simulink model "AcasXuClosedLoop_m_1"  (R2019b)
settings: Solver=VariableStepAuto  StartTime=0.0  StopTime=30  RelTol=1e-3
libraries: neural x1560, simulink x2
(part 3 of 85)

== system AcasXuClosedLoop_m_1/networks/AcasXu_2_1/Process Output 1 ==
  a : Inport  PortDimensions=5
      mask Display: e = 0.06;c1 = [120 230 180]/255;c2 = ([120 230 180]+0)/(256+128);c3 = ([120 230 180]+128)/(256+128);patch([0 1 1 0],[0 0 1 1],c1);patch([0 1 1 1-e 1-e 0+e],[0 0 1 1-e 0+e 0+e],c2);patch([0 0 1 1-e 0+e 0+e],[0 1 1 1-e 1-e 0+e],c3);plot([0 1 1 0 0],[0 0 1 1 0]);
  y : Outport  PortDimensions=5
      mask Display: e = 0.06;c1 = [120 230 180]/255;c2 = ([120 230 180]+0)/(256+128);c3 = ([120 230 180]+128)/(256+128);patch([0 1 1 0],[0 0 1 1],c1);patch([0 1 1 1-e 1-e 0+e],[0 0 1 1-e 0+e 0+e],c2);patch([0 0 1 1-e 0+e 0+e],[0 1 1 1-e 1-e 0+e],c3);plot([0 1 1 0 0],[0 0 1 1 0]);
  wires:
  a/1 -> y/1

== system AcasXuClosedLoop_m_1/networks/AcasXu_3_1/Layer 1 ==
  "p{1}" : Inport  PortDimensions=5
      mask Display: e = 0.06;c1 = [120 230 180]/255;c2 = ([120 230 180]+0)/(256+128);c3 = ([120 230 180]+128)/(256+128);patch([0 1 1 0],[0 0 1 1],c1);patch([0 1 1 1-e 1-e 0+e],[0 0 1 1-e 0+e 0+e],c2);patch([0 0 1 1-e 0+e 0+e],[0 1 1 1-e 1-e 0+e],c3);plot([0 1 1 0 0],[0 0 1 1 0]);
  Delays 1 : Subsystem
      mask Display: e = 0.06;c1 = [120 150 230]/255;c2 = ([120 150 230]+0)/383;c3 = ([120 150 230]+128)/383;patch([0 1 1 0],[0 0 1 1],c1);patch([0 1 1 1-e 1-e 0+e],[0 0 1 1-e 0+e 0+e],c2);patch([0 0 1 1-e 0+e 0+e],[0 1 1 1-e 1-e 0+e],c3);plot([0 1 1 0 0],[0 0 1 1 0]);disp('0');
  "IW{1,1}" : Subsystem
      mask Display: e = 0.06;c1 = [120 150 230]/255;c2 = ([120 150 230]+0)/383;c3 = ([120 150 230]+128)/383;patch([0 1 1 0],[0 0 1 1],c1);patch([0 1 1 1-e 1-e 0+e],[0 0 1 1-e 0+e 0+e],c2);patch([0 0 1 1-e 0+e 0+e],[0 1 1 1-e 1-e 0+e],c3);plot([0 1 1 0 0],[0 0 1 1 0]);disp('W');
  "b{1}" : Constant  Value=[-0.63411600000000001298161578233703039586544036865234375;-0.86285800000000001386268877467955462634563446044921875;0.0263649000000000001409095062854248681105673313140869140625;-0.77790700000000001512745484433253295719623565673828125;-0.172433000000000002938094212368014268577098846435546875;0.08491990000000000649027498411669512279331684112548828125;0.2125950000000000061906035853098728694021701812744140625;-0.0674716999999999955672791429606149904429912567138671875;-0.37667200000000000681410483593936078250408172607421875;0.2037360000000000004316547119742608629167079925537109375;0.1262359999999999871089784164723823778331279754638671875;-0.5560300000000000242295072894194163382053375244140625;-0.45896700000000001384847791996435262262821197509765625;-0.306524000000000018673063095775432884693145751953125;-0.06648220000000000518003417937507038004696369171142578125;-0.53795800000000004725819735540426336228847503662109375;0.3475610000000000088249407781404443085193634033203125;-0.0226518999999999991190602344204307883046567440032958984375;-0.387670000000000014583889651476056315004825592041015625;-0.5660089999999999843538489585625939071178436279296875;-0.072275699999999998279776036724797450006008148193359375;0.1934430000000000038351544162651407532393932342529296875;0.16017300000000000981259518084698356688022613525390625;-0.11682399999999999729016764149491791613399982452392578125;0.0849908000000000052320814347694977186620235443115234375;-0.0176456000000000008676170892840673332102596759796142578125;-0.19644600000000000949995637711253948509693145751953125;0.193624999999999991562305012848810292780399322509765625;-0.6789519999999999999573674358543939888477325439453125;-0.045666199999999997072297475142477196641266345977783203125;0.1721910000000000107167608121017110534012317657470703125;-0.36496099999999997987032429591636173427104949951171875;-0.34974600000000000132871491587138734757900238037109375;-0.56786199999999997789501549050328321754932403564453125;-0.770345999999999975216269376687705516815185546875;-0.10563799999999999579269882588050677441060543060302734375;-0.82683600000000001539746108392137102782726287841796875;0.5441249999999999698019337301957421004772186279296875;0.552065999999999945657691569067537784576416015625;-0.279227999999999976221687347788247279822826385498046875;-0.0244107999999999998597122186083652195520699024200439453125;-0.6494180000000000507753838974167592823505401611328125;-0.67569800000000002082600758512853644788265228271484375;-0.0534702999999999983860021757209324277937412261962890625;0.043996899999999998509547793901219847612082958221435546875;-0.10106999999999999317878973670303821563720703125;0.10270100000000000062261307220978778786957263946533203125;0.385166999999999981607601284849806688725948333740234375;-0.642935000000000034248159863636828958988189697265625;-0.0231879000000000008718803456986279343254864215850830078125]
      mask Display: e = 0.06;c1 = [120 150 230]/255;c2 = ([120 150 230]+0)/383;c3 = ([120 150 230]+128)/383;patch([0 1 1 0],[0 0 1 1],c1);patch([0 1 1 1-e 1-e 0+e],[0 0 1 1-e 0+e 0+e],c2);patch([0 0 1 1-e 0+e 0+e],[0 1 1 1-e 1-e 0+e],c3);plot([0 1 1 0 0],[0 0 1 1 0]);disp('b');
  netsum : Sum  Inputs=2  SaturateOnIntegerOverflow=on  InputSameDT=on  OutDataTypeStr=Inherit: Same as first input
      mask Display: e = 0.06;c1 = [120 150 230]/255;c2 = ([120 150 230]+0)/383;c3 = ([120 150 230]+128)/383;patch([0 1 1 0],[0 0 1 1],c1);patch([0 1 1 1-e 1-e 0+e],[0 0 1 1-e 0+e 0+e],c2);patch([0 0 1 1-e 0+e 0+e],[0 1 1 1-e 1-e 0+e],c3);plot([0 1 1 0 0],[0 0 1 1 0]);disp('+');
  tansig : neural/Transfer Functions/tansig
      settings: SourceProductName=Deep Learning Toolbox
  "a{1}" : Outport  InitialOutput=[0;0;0;0;0;0;0;0;0;0;0;0;0;0;0;0;0;0;0;0;0;0;0;0;0;0;0;0;0;0;0;0;0;0;0;0;0;0;0;0;0;0;0;0;0;0;0;0;0;0]
      mask Display: e = 0.06;c1 = [120 230 180]/255;c2 = ([120 230 180]+0)/(256+128);c3 = ([120 230 180]+128)/(256+128);patch([0 1 1 0],[0 0 1 1],c1);patch([0 1 1 1-e 1-e 0+e],[0 0 1 1-e 0+e 0+e],c2);patch([0 0 1 1-e 0+e 0+e],[0 1 1 1-e 1-e 0+e],c3);plot([0 1 1 0 0],[0 0 1 1 0]);
  wires:
  tansig/1 -> "a{1}"/1
  netsum/1 -> tansig/1
  "b{1}"/1 -> netsum/2
  "IW{1,1}"/1("iz{1,1}") -> netsum/1
  Delays 1/1("pd{1,1}") -> "IW{1,1}"/1("pd{1,1}")
  "p{1}"/1 -> Delays 1/1("p{1}")

== system AcasXuClosedLoop_m_1/networks/AcasXu_3_1/Layer 2 ==
  "a{1} " : Inport  PortDimensions=50
      mask Display: e = 0.06;c1 = [120 230 180]/255;c2 = ([120 230 180]+0)/(256+128);c3 = ([120 230 180]+128)/(256+128);patch([0 1 1 0],[0 0 1 1],c1);patch([0 1 1 1-e 1-e 0+e],[0 0 1 1-e 0+e 0+e],c2);patch([0 0 1 1-e 0+e 0+e],[0 1 1 1-e 1-e 0+e],c3);plot([0 1 1 0 0],[0 0 1 1 0]);
  Delays 1 : Subsystem
      mask Display: e = 0.06;c1 = [120 150 230]/255;c2 = ([120 150 230]+0)/383;c3 = ([120 150 230]+128)/383;patch([0 1 1 0],[0 0 1 1],c1);patch([0 1 1 1-e 1-e 0+e],[0 0 1 1-e 0+e 0+e],c2);patch([0 0 1 1-e 0+e 0+e],[0 1 1 1-e 1-e 0+e],c3);plot([0 1 1 0 0],[0 0 1 1 0]);disp('0');
  "LW{2,1}" : Subsystem
      mask Display: e = 0.06;c1 = [120 150 230]/255;c2 = ([120 150 230]+0)/383;c3 = ([120 150 230]+128)/383;patch([0 1 1 0],[0 0 1 1],c1);patch([0 1 1 1-e 1-e 0+e],[0 0 1 1-e 0+e 0+e],c2);patch([0 0 1 1-e 0+e 0+e],[0 1 1 1-e 1-e 0+e],c3);plot([0 1 1 0 0],[0 0 1 1 0]);disp('W');
  "b{2}" : Constant  Value=[-0.421233000000000024076740601230994798243045806884765625;0.1434140000000000136903821612577303312718868255615234375;-0.99709400000000003583267016438185237348079681396484375;0.377188000000000023259616455106879584491252899169921875;-0.01035819999999999969919617370806008693762123584747314453125;-0.71935300000000002018651912294444628059864044189453125;-0.334293000000000006810552122260560281574726104736328125;-0.773163999999999962398078423575498163700103759765625;-0.003741040000000000163848934420229852548800408840179443359375;-0.0589896000000000031437963343705632723867893218994140625;-0.35057199999999999473487832801765762269496917724609375;-0.91174900000000003164046802339726127684116363525390625;-0.57765400000000000080291329140891321003437042236328125;-1.0581300000000000149924517245381139218807220458984375;0.278627000000000013546497257266310043632984161376953125;-0.0093275500000000004241496043277948047034442424774169921875;-0.0123510000000000008668621376273222267627716064453125;-0.404268000000000016225243371081887744367122650146484375;-0.746971999999999969332975524594075977802276611328125;-0.08297960000000000058140159353570197708904743194580078125;-1.167079999999999895266000748961232602596282958984375;-0.5178279999999999549942231169552542269229888916015625;0.68078300000000002700772938624140806496143341064453125;-0.2080639999999999989466203942356514744460582733154296875;-0.80007799999999995588240153665537945926189422607421875;5.53026000000000013986749258787511962509597651660442352294921875e-05;-0.1960199999999999997957189634689711965620517730712890625;0.600638000000000005229594535194337368011474609375;0.28952699999999997881872104699141345918178558349609375;0.48111599999999998811262003073352389037609100341796875;0.028625799999999999856381549534489749930799007415771484375;0.255568999999999990624388601645478047430515289306640625;-0.00619316999999999957815521867132702027447521686553955078125;-0.7419949999999999601385525238583795726299285888671875;-0.1441759999999999986020071673920028842985630035400390625;-0.556777999999999995139887687400914728641510009765625;-0.2580999999999999960920149533194489777088165283203125;-0.282907999999999992812860227786586619913578033447265625;-0.48276499999999999968025576890795491635799407958984375;-0.004546970000000000004802824804528427193872630596160888671875;0.302254999999999995896615700985421426594257354736328125;-0.6570489999999999941593387120519764721393585205078125;-0.5748919999999999586037802146165631711483001708984375;1.2579299999999999926103555480949580669403076171875;0.222015999999999991132426657713949680328369140625;1.349930000000000074322770160506479442119598388671875;-0.423561000000000020815349444092134945094585418701171875;-0.427883000000000013329781722859479486942291259765625;0.304840999999999973102404737801407463848590850830078125;-0.10981899999999999995026200849679298698902130126953125]
      mask Display: e = 0.06;c1 = [120 150 230]/255;c2 = ([120 150 230]+0)/383;c3 = ([120 150 230]+128)/383;patch([0 1 1 0],[0 0 1 1],c1);patch([0 1 1 1-e 1-e 0+e],[0 0 1 1-e 0+e 0+e],c2);patch([0 0 1 1-e 0+e 0+e],[0 1 1 1-e 1-e 0+e],c3);plot([0 1 1 0 0],[0 0 1 1 0]);disp('b');
  netsum : Sum  Inputs=2  SaturateOnIntegerOverflow=on  InputSameDT=on  OutDataTypeStr=Inherit: Same as first input
      mask Display: e = 0.06;c1 = [120 150 230]/255;c2 = ([120 150 230]+0)/383;c3 = ([120 150 230]+128)/383;patch([0 1 1 0],[0 0 1 1],c1);patch([0 1 1 1-e 1-e 0+e],[0 0 1 1-e 0+e 0+e],c2);patch([0 0 1 1-e 0+e 0+e],[0 1 1 1-e 1-e 0+e],c3);plot([0 1 1 0 0],[0 0 1 1 0]);disp('+');
  tansig : neural/Transfer Functions/tansig
      settings: SourceProductName=Deep Learning Toolbox
  "a{2}" : Outport  InitialOutput=[0;0;0;0;0;0;0;0;0;0;0;0;0;0;0;0;0;0;0;0;0;0;0;0;0;0;0;0;0;0;0;0;0;0;0;0;0;0;0;0;0;0;0;0;0;0;0;0;0;0]
      mask Display: e = 0.06;c1 = [120 230 180]/255;c2 = ([120 230 180]+0)/(256+128);c3 = ([120 230 180]+128)/(256+128);patch([0 1 1 0],[0 0 1 1],c1);patch([0 1 1 1-e 1-e 0+e],[0 0 1 1-e 0+e 0+e],c2);patch([0 0 1 1-e 0+e 0+e],[0 1 1 1-e 1-e 0+e],c3);plot([0 1 1 0 0],[0 0 1 1 0]);
  wires:
  tansig/1 -> "a{2}"/1
  netsum/1 -> tansig/1
  "b{2}"/1 -> netsum/2
  "LW{2,1}"/1("lz{2,1}") -> netsum/1
  Delays 1/1("pd{2,1}") -> "LW{2,1}"/1("ad{2,1}")
  "a{1} "/1 -> Delays 1/1("p{2}")

== system AcasXuClosedLoop_m_1/networks/AcasXu_3_1/Layer 3 ==
  "a{2} " : Inport  PortDimensions=50
      mask Display: e = 0.06;c1 = [120 230 180]/255;c2 = ([120 230 180]+0)/(256+128);c3 = ([120 230 180]+128)/(256+128);patch([0 1 1 0],[0 0 1 1],c1);patch([0 1 1 1-e 1-e 0+e],[0 0 1 1-e 0+e 0+e],c2);patch([0 0 1 1-e 0+e 0+e],[0 1 1 1-e 1-e 0+e],c3);plot([0 1 1 0 0],[0 0 1 1 0]);
  Delays 1 : Subsystem
      mask Display: e = 0.06;c1 = [120 150 230]/255;c2 = ([120 150 230]+0)/383;c3 = ([120 150 230]+128)/383;patch([0 1 1 0],[0 0 1 1],c1);patch([0 1 1 1-e 1-e 0+e],[0 0 1 1-e 0+e 0+e],c2);patch([0 0 1 1-e 0+e 0+e],[0 1 1 1-e 1-e 0+e],c3);plot([0 1 1 0 0],[0 0 1 1 0]);disp('0');
  "LW{3,2}" : Subsystem
      mask Display: e = 0.06;c1 = [120 150 230]/255;c2 = ([120 150 230]+0)/383;c3 = ([120 150 230]+128)/383;patch([0 1 1 0],[0 0 1 1],c1);patch([0 1 1 1-e 1-e 0+e],[0 0 1 1-e 0+e 0+e],c2);patch([0 0 1 1-e 0+e 0+e],[0 1 1 1-e 1-e 0+e],c3);plot([0 1 1 0 0],[0 0 1 1 0]);disp('W');
  "b{3}" : Constant  Value=[1.0556000000000000937916411203332245349884033203125;-1.4562500000000000444089209850062616169452667236328125;0.35456500000000001904254531837068498134613037109375;-0.37268800000000001926281356645631603896617889404296875;1.9437599999999999322852772820624522864818572998046875;0.485267999999999977145392904276377521455287933349609375;-0.03026600000000000123545618180287419818341732025146484375;0.1490809999999999913011805574569734744727611541748046875;-1.6594700000000000006394884621840901672840118408203125;1.188099999999999933919525574310682713985443115234375;-1.2918600000000000083133500083931721746921539306640625;-0.263782000000000016459722473882720805704593658447265625;-0.73707800000000001094946355806314386427402496337890625;-0.85128499999999995839772282124613411724567413330078125;0.11599900000000000488409312993098865263164043426513671875;-0.062371299999999997576427546164268278516829013824462890625;-0.032435600000000001930100523850342142395675182342529296875;0.269172000000000022357227180691552348434925079345703125;-0.1436570000000000069118044621063745580613613128662109375;0.1983350000000000112887477143885917030274868011474609375;-1.749470000000000080575546235195361077785491943359375;-0.259944000000000008387956995647982694208621978759765625;-0.6662820000000000408846290156361646950244903564453125;0.1677220000000000099671382258748053573071956634521484375;-0.40030500000000002192024339819909073412418365478515625;-0.58646100000000001006839056572061963379383087158203125;-0.0123961999999999995802912877707058214582502841949462890625;-0.27758599999999999941024952931911684572696685791015625;0.322699000000000013610446103484719060361385345458984375;0.289306000000000007599254558954271487891674041748046875;-0.0636571999999999971198150205964338965713977813720703125;0.07619430000000000646753761657237191684544086456298828125;-0.26723200000000002507505314497393555939197540283203125;-0.886967999999999978655296217766590416431427001953125;0.074126899999999995571897670743055641651153564453125;-0.60304100000000004921929530610213987529277801513671875;-1.47614000000000000767386154620908200740814208984375;-0.99038400000000004208544623907073400914669036865234375;0.2862970000000000236894948102417401969432830810546875;0.01722970000000000057038818113142042420804500579833984375;-0.0288367999999999992388755032379776821471750736236572265625;0.55647699999999999942446038403431884944438934326171875;0.350275999999999976264319911933853290975093841552734375;-2.10245000000000015205614545266143977642059326171875;-0.0292092000000000011350476114557750406675040721893310546875;0.05668299999999999727595678677971591241657733917236328125;-0.7748880000000000212168060897965915501117706298828125;-0.030838999999999998358202191184318508021533489227294921875;-0.3683710000000000039932501749717630445957183837890625;-0.0617846999999999979547027351145516149699687957763671875]
      mask Display: e = 0.06;c1 = [120 150 230]/255;c2 = ([120 150 230]+0)/383;c3 = ([120 150 230]+128)/383;patch([0 1 1 0],[0 0 1 1],c1);patch([0 1 1 1-e 1-e 0+e],[0 0 1 1-e 0+e 0+e],c2);patch([0 0 1 1-e 0+e 0+e],[0 1 1 1-e 1-e 0+e],c3);plot([0 1 1 0 0],[0 0 1 1 0]);disp('b');
  netsum : Sum  Inputs=2  SaturateOnIntegerOverflow=on  InputSameDT=on  OutDataTypeStr=Inherit: Same as first input
      mask Display: e = 0.06;c1 = [120 150 230]/255;c2 = ([120 150 230]+0)/383;c3 = ([120 150 230]+128)/383;patch([0 1 1 0],[0 0 1 1],c1);patch([0 1 1 1-e 1-e 0+e],[0 0 1 1-e 0+e 0+e],c2);patch([0 0 1 1-e 0+e 0+e],[0 1 1 1-e 1-e 0+e],c3);plot([0 1 1 0 0],[0 0 1 1 0]);disp('+');
  tansig : neural/Transfer Functions/tansig
      settings: SourceProductName=Deep Learning Toolbox
  "a{3}" : Outport  InitialOutput=[0;0;0;0;0;0;0;0;0;0;0;0;0;0;0;0;0;0;0;0;0;0;0;0;0;0;0;0;0;0;0;0;0;0;0;0;0;0;0;0;0;0;0;0;0;0;0;0;0;0]
      mask Display: e = 0.06;c1 = [120 230 180]/255;c2 = ([120 230 180]+0)/(256+128);c3 = ([120 230 180]+128)/(256+128);patch([0 1 1 0],[0 0 1 1],c1);patch([0 1 1 1-e 1-e 0+e],[0 0 1 1-e 0+e 0+e],c2);patch([0 0 1 1-e 0+e 0+e],[0 1 1 1-e 1-e 0+e],c3);plot([0 1 1 0 0],[0 0 1 1 0]);
  wires:
  tansig/1 -> "a{3}"/1
  netsum/1 -> tansig/1
  "b{3}"/1 -> netsum/2
  "LW{3,2}"/1("lz{3,2}") -> netsum/1
  Delays 1/1("pd{3,2}") -> "LW{3,2}"/1("ad{3,2}")
  "a{2} "/1 -> Delays 1/1("p{3}")

== system AcasXuClosedLoop_m_1/networks/AcasXu_3_1/Layer 4 ==
  "a{3} " : Inport  PortDimensions=50
      mask Display: e = 0.06;c1 = [120 230 180]/255;c2 = ([120 230 180]+0)/(256+128);c3 = ([120 230 180]+128)/(256+128);patch([0 1 1 0],[0 0 1 1],c1);patch([0 1 1 1-e 1-e 0+e],[0 0 1 1-e 0+e 0+e],c2);patch([0 0 1 1-e 0+e 0+e],[0 1 1 1-e 1-e 0+e],c3);plot([0 1 1 0 0],[0 0 1 1 0]);
  Delays 1 : Subsystem
      mask Display: e = 0.06;c1 = [120 150 230]/255;c2 = ([120 150 230]+0)/383;c3 = ([120 150 230]+128)/383;patch([0 1 1 0],[0 0 1 1],c1);patch([0 1 1 1-e 1-e 0+e],[0 0 1 1-e 0+e 0+e],c2);patch([0 0 1 1-e 0+e 0+e],[0 1 1 1-e 1-e 0+e],c3);plot([0 1 1 0 0],[0 0 1 1 0]);disp('0');
  "LW{4,3}" : Subsystem
      mask Display: e = 0.06;c1 = [120 150 230]/255;c2 = ([120 150 230]+0)/383;c3 = ([120 150 230]+128)/383;patch([0 1 1 0],[0 0 1 1],c1);patch([0 1 1 1-e 1-e 0+e],[0 0 1 1-e 0+e 0+e],c2);patch([0 0 1 1-e 0+e 0+e],[0 1 1 1-e 1-e 0+e],c3);plot([0 1 1 0 0],[0 0 1 1 0]);disp('W');
  "b{4}" : Constant  Value=[0.1965349999999999874855660664252354763448238372802734375;-0.39496500000000001051603248924948275089263916015625;0.0831124000000000029420021974146948195993900299072265625;-0.8129589999999999871960199016029946506023406982421875;-0.267452999999999996294519633011077530682086944580078125;-0.62282899999999996598631923916400410234928131103515625;-0.5259570000000000078443918027915060520172119140625;0.16539300000000001222844048243132419884204864501953125;-1.460080000000000044479975258582271635532379150390625;2.108870000000000022311041902867145836353302001953125;-0.7184180000000000010373923942097462713718414306640625;0.334618999999999999772626324556767940521240234375;-0.0290208999999999987806642565146830747835338115692138671875;-1.4232800000000001006128513836301863193511962890625;0.1955969999999999930917482515724259428679943084716796875;0.2019459999999999866293620698343147523701190948486328125;-1.14275999999999999801048033987171947956085205078125;2.440440000000000164703806149191223084926605224609375;-0.0841351999999999933255168116374989040195941925048828125;-1.0137799999999999034372422102023847401142120361328125;0.919775000000000009237055564881302416324615478515625;-1.3366100000000000758149099056026898324489593505859375;-2.752540000000000208757455766317434608936309814453125;-0.10592500000000000526245713672324200160801410675048828125;-0.97771799999999997599076095866621471941471099853515625;0.3647489999999999898960822974913753569126129150390625;0.9579910000000000369624331142404116690158843994140625;-0.467220000000000024176216584237408824265003204345703125;0.09166290000000000548485701301615335978567600250244140625;-1.423890000000000100044417195022106170654296875;-1.8000700000000000589039927945123054087162017822265625;0.9487229999999999829896069059032015502452850341796875;-0.197079000000000004177991286269389092922210693359375;0.6932519999999999793516280988114885985851287841796875;-1.2097599999999999464961319972644560039043426513671875;-1.24059000000000008157030606525950133800506591796875;-0.63907999999999998141930745987338013947010040283203125;0.0181432000000000016870504992994028725661337375640869140625;-0.2202240000000000030855318300382350571453571319580078125;-1.83692000000000010828671292983926832675933837890625;2.902439999999999908908421275555156171321868896484375;0.259921999999999986386001182836480438709259033203125;0.74938099999999996381205846773809753358364105224609375;0.0329962000000000033050895353881060145795345306396484375;0.0563639999999999974367170807454385794699192047119140625;-1.997370000000000089812601800076663494110107421875;-0.378624999999999989341858963598497211933135986328125;0.5712930000000000507753838974167592823505401611328125;1.9845200000000000617461637375527061522006988525390625;0.39603500000000002589928271845565177500247955322265625]
      mask Display: e = 0.06;c1 = [120 150 230]/255;c2 = ([120 150 230]+0)/383;c3 = ([120 150 230]+128)/383;patch([0 1 1 0],[0 0 1 1],c1);patch([0 1 1 1-e 1-e 0+e],[0 0 1 1-e 0+e 0+e],c2);patch([0 0 1 1-e 0+e 0+e],[0 1 1 1-e 1-e 0+e],c3);plot([0 1 1 0 0],[0 0 1 1 0]);disp('b');
  netsum : Sum  Inputs=2  SaturateOnIntegerOverflow=on  InputSameDT=on  OutDataTypeStr=Inherit: Same as first input
      mask Display: e = 0.06;c1 = [120 150 230]/255;c2 = ([120 150 230]+0)/383;c3 = ([120 150 230]+128)/383;patch([0 1 1 0],[0 0 1 1],c1);patch([0 1 1 1-e 1-e 0+e],[0 0 1 1-e 0+e 0+e],c2);patch([0 0 1 1-e 0+e 0+e],[0 1 1 1-e 1-e 0+e],c3);plot([0 1 1 0 0],[0 0 1 1 0]);disp('+');
  tansig : neural/Transfer Functions/tansig
      settings: SourceProductName=Deep Learning Toolbox
  "a{4}" : Outport  InitialOutput=[0;0;0;0;0;0;0;0;0;0;0;0;0;0;0;0;0;0;0;0;0;0;0;0;0;0;0;0;0;0;0;0;0;0;0;0;0;0;0;0;0;0;0;0;0;0;0;0;0;0]
      mask Display: e = 0.06;c1 = [120 230 180]/255;c2 = ([120 230 180]+0)/(256+128);c3 = ([120 230 180]+128)/(256+128);patch([0 1 1 0],[0 0 1 1],c1);patch([0 1 1 1-e 1-e 0+e],[0 0 1 1-e 0+e 0+e],c2);patch([0 0 1 1-e 0+e 0+e],[0 1 1 1-e 1-e 0+e],c3);plot([0 1 1 0 0],[0 0 1 1 0]);
  wires:
  tansig/1 -> "a{4}"/1
  netsum/1 -> tansig/1
  "b{4}"/1 -> netsum/2
  "LW{4,3}"/1("lz{4,3}") -> netsum/1
  Delays 1/1("pd{4,3}") -> "LW{4,3}"/1("ad{4,3}")
  "a{3} "/1 -> Delays 1/1("p{4}")

== system AcasXuClosedLoop_m_1/networks/AcasXu_3_1/Layer 5 ==
  "a{4} " : Inport  PortDimensions=50
      mask Display: e = 0.06;c1 = [120 230 180]/255;c2 = ([120 230 180]+0)/(256+128);c3 = ([120 230 180]+128)/(256+128);patch([0 1 1 0],[0 0 1 1],c1);patch([0 1 1 1-e 1-e 0+e],[0 0 1 1-e 0+e 0+e],c2);patch([0 0 1 1-e 0+e 0+e],[0 1 1 1-e 1-e 0+e],c3);plot([0 1 1 0 0],[0 0 1 1 0]);
  Delays 1 : Subsystem
      mask Display: e = 0.06;c1 = [120 150 230]/255;c2 = ([120 150 230]+0)/383;c3 = ([120 150 230]+128)/383;patch([0 1 1 0],[0 0 1 1],c1);patch([0 1 1 1-e 1-e 0+e],[0 0 1 1-e 0+e 0+e],c2);patch([0 0 1 1-e 0+e 0+e],[0 1 1 1-e 1-e 0+e],c3);plot([0 1 1 0 0],[0 0 1 1 0]);disp('0');
  "LW{5,4}" : Subsystem
      mask Display: e = 0.06;c1 = [120 150 230]/255;c2 = ([120 150 230]+0)/383;c3 = ([120 150 230]+128)/383;patch([0 1 1 0],[0 0 1 1],c1);patch([0 1 1 1-e 1-e 0+e],[0 0 1 1-e 0+e 0+e],c2);patch([0 0 1 1-e 0+e 0+e],[0 1 1 1-e 1-e 0+e],c3);plot([0 1 1 0 0],[0 0 1 1 0]);disp('W');
  "b{5}" : Constant  Value=[0.47812900000000002620481609483249485492706298828125;0.51515699999999997604760437752702273428440093994140625;0.41300199999999998023980651851161383092403411865234375;-0.6262309999999999821085339135606773197650909423828125;-0.059302399999999998170263637575772008858621120452880859375;-0.10103700000000000180921944092915509827435016632080078125;-2.115899999999999891997504164464771747589111328125;0.53538399999999997103117266306071542203426361083984375;0.6186760000000000037090330806677229702472686767578125;1.745670000000000054996007747831754386425018310546875;0.259404000000000023451462993762106634676456451416015625;1.3870199999999999196376165855326689779758453369140625;-1.7769399999999999639754832969629205763339996337890625;0.360806000000000015592860336255398578941822052001953125;-0.92147900000000004805400521945557557046413421630859375;-1.058710000000000039932501749717630445957183837890625;-0.0424293000000000031235458664014004170894622802734375;0.40383599999999997276489693831535987555980682373046875;0.399467000000000016513013179064728319644927978515625;0.08201920000000000043893777501580188982188701629638671875;-0.84730199999999999960209606797434389591217041015625;-0.26574500000000000898836560736526735126972198486328125;0.461569999999999980300202651051222346723079681396484375;1.4558199999999998919264498908887617290019989013671875;1.0840899999999999980815346134477294981479644775390625;-1.4489199999999999857180910112219862639904022216796875;-0.68995799999999996021671222479199059307575225830078125;0.446290000000000020019541580040822736918926239013671875;0.98659799999999997499600112860207445919513702392578125;-0.288679999999999992166266338244895450770854949951171875;0.93531500000000000749622586226905696094036102294921875;1.21314000000000010714984455262310802936553955078125;-0.4377159999999999939745976007543504238128662109375;1.1303199999999999914024328973027877509593963623046875;-0.07310049999999999881250545286093256436288356781005859375;-0.254632000000000024986235303003923036158084869384765625;-0.417215999999999975766939996901783160865306854248046875;0.2296870000000000022755131112717208452522754669189453125;0.197593999999999991867838389225653372704982757568359375;0.77214799999999994550847759455791674554347991943359375;-0.12305800000000000071764816311770118772983551025390625;1.1698100000000000164845914696343243122100830078125;0.386216999999999976989073502409155480563640594482421875;-0.2494929999999999925552884860735503025352954864501953125;-0.6158010000000000427888835474732331931591033935546875;-1.6749099999999998988897687013377435505390167236328125;1.7169200000000000017053025658242404460906982421875;1.1729600000000000026290081223123706877231597900390625;0.430236000000000007315037464650231413543224334716796875;-0.63865300000000002622613237690529786050319671630859375]
      mask Display: e = 0.06;c1 = [120 150 230]/255;c2 = ([120 150 230]+0)/383;c3 = ([120 150 230]+128)/383;patch([0 1 1 0],[0 0 1 1],c1);patch([0 1 1 1-e 1-e 0+e],[0 0 1 1-e 0+e 0+e],c2);patch([0 0 1 1-e 0+e 0+e],[0 1 1 1-e 1-e 0+e],c3);plot([0 1 1 0 0],[0 0 1 1 0]);disp('b');
  netsum : Sum  Inputs=2  SaturateOnIntegerOverflow=on  InputSameDT=on  OutDataTypeStr=Inherit: Same as first input
      mask Display: e = 0.06;c1 = [120 150 230]/255;c2 = ([120 150 230]+0)/383;c3 = ([120 150 230]+128)/383;patch([0 1 1 0],[0 0 1 1],c1);patch([0 1 1 1-e 1-e 0+e],[0 0 1 1-e 0+e 0+e],c2);patch([0 0 1 1-e 0+e 0+e],[0 1 1 1-e 1-e 0+e],c3);plot([0 1 1 0 0],[0 0 1 1 0]);disp('+');
  tansig : neural/Transfer Functions/tansig
      settings: SourceProductName=Deep Learning Toolbox
  "a{5}" : Outport  InitialOutput=[0;0;0;0;0;0;0;0;0;0;0;0;0;0;0;0;0;0;0;0;0;0;0;0;0;0;0;0;0;0;0;0;0;0;0;0;0;0;0;0;0;0;0;0;0;0;0;0;0;0]
      mask Display: e = 0.06;c1 = [120 230 180]/255;c2 = ([120 230 180]+0)/(256+128);c3 = ([120 230 180]+128)/(256+128);patch([0 1 1 0],[0 0 1 1],c1);patch([0 1 1 1-e 1-e 0+e],[0 0 1 1-e 0+e 0+e],c2);patch([0 0 1 1-e 0+e 0+e],[0 1 1 1-e 1-e 0+e],c3);plot([0 1 1 0 0],[0 0 1 1 0]);
  wires:
  tansig/1 -> "a{5}"/1
  netsum/1 -> tansig/1
  "b{5}"/1 -> netsum/2
  "LW{5,4}"/1("lz{5,4}") -> netsum/1
  Delays 1/1("pd{5,4}") -> "LW{5,4}"/1("ad{5,4}")
  "a{4} "/1 -> Delays 1/1("p{5}")

== system AcasXuClosedLoop_m_1/networks/AcasXu_3_1/Layer 6 ==
  "a{5} " : Inport  PortDimensions=50
      mask Display: e = 0.06;c1 = [120 230 180]/255;c2 = ([120 230 180]+0)/(256+128);c3 = ([120 230 180]+128)/(256+128);patch([0 1 1 0],[0 0 1 1],c1);patch([0 1 1 1-e 1-e 0+e],[0 0 1 1-e 0+e 0+e],c2);patch([0 0 1 1-e 0+e 0+e],[0 1 1 1-e 1-e 0+e],c3);plot([0 1 1 0 0],[0 0 1 1 0]);
  Delays 1 : Subsystem
      mask Display: e = 0.06;c1 = [120 150 230]/255;c2 = ([120 150 230]+0)/383;c3 = ([120 150 230]+128)/383;patch([0 1 1 0],[0 0 1 1],c1);patch([0 1 1 1-e 1-e 0+e],[0 0 1 1-e 0+e 0+e],c2);patch([0 0 1 1-e 0+e 0+e],[0 1 1 1-e 1-e 0+e],c3);plot([0 1 1 0 0],[0 0 1 1 0]);disp('0');
  "LW{6,5}" : Subsystem
      mask Display: e = 0.06;c1 = [120 150 230]/255;c2 = ([120 150 230]+0)/383;c3 = ([120 150 230]+128)/383;patch([0 1 1 0],[0 0 1 1],c1);patch([0 1 1 1-e 1-e 0+e],[0 0 1 1-e 0+e 0+e],c2);patch([0 0 1 1-e 0+e 0+e],[0 1 1 1-e 1-e 0+e],c3);plot([0 1 1 0 0],[0 0 1 1 0]);disp('W');
  "b{6}" : Constant  Value=[-0.308194999999999996731503415503539144992828369140625;-0.5165889999999999648849779987358488142490386962890625;-0.0212764000000000008672174089952022768557071685791015625;-0.09961119999999999696793651082771248184144496917724609375;-0.10795399999999999440802866956801153719425201416015625;0.012656699999999999894928492949475185014307498931884765625;-0.95685600000000003984013119406881742179393768310546875;-0.0758999999999999952482454546043300069868564605712890625;-0.392367999999999994553689930398832075297832489013671875;-0.55846399999999996044408590023522265255451202392578125;-0.090985499999999996934008095195167697966098785400390625;-0.94885399999999997522337480404530651867389678955078125;-0.166198000000000012388312597977346740663051605224609375;-0.1367629999999999956816765234179911203682422637939453125;-0.003977320000000000334294814052782385260798037052154541015625;-0.01260509999999999929121141661880756146274507045745849609375;-0.018286299999999998389110800189882866106927394866943359375;-0.8251049999999999773336867292528040707111358642578125;0.03823780000000000234283703548499033786356449127197265625;-0.264390999999999987135623769063386134803295135498046875;-0.069768200000000002436451040921383537352085113525390625;0.0112919999999999999540367667805185192264616489410400390625;-0.0174611999999999996380228850512139615602791309356689453125;-0.0031774400000000001254019110774606815539300441741943359375;-0.281694999999999973194775293450220488011837005615234375;-0.6130539999999999878355083637870848178863525390625;0.498057000000000027473134878164273686707019805908203125;-0.051213899999999999701483233138787909410893917083740234375;-0.047606500000000002981170865723470342345535755157470703125;-0.000580838999999999986388610206944349556579254567623138427734375;-0.000924406000000000012406520255581199307925999164581298828125;-0.06332469999999999765716296451500966213643550872802734375;-0.06918459999999999887609902771146153099834918975830078125;-0.1222820000000000018047785488306544721126556396484375;-0.77860099999999998754418584212544374167919158935546875;-0.0016212200000000000395250498996801979956217110157012939453125;0.107453999999999993963939459717948921024799346923828125;-0.297453000000000022939872224014834500849246978759765625;0.6060090000000000198809857465676032006740570068359375;0.06889030000000000153459467355787637643516063690185546875;-0.59869600000000000594724269831203855574131011962890625;-0.2253509999999999957598362243516021408140659332275390625;0.06327660000000000228848051619934267364442348480224609375;-0.262585000000000012843059948863810859620571136474609375;-0.83241799999999999126742977750836871564388275146484375;-0.450313000000000018818724356606253422796726226806640625;-0.5228120000000000544559952686540782451629638671875;-0.1568219999999999891837632048918749205768108367919921875;-1.2062299999999999133848405108437873423099517822265625;-0.0017704299999999999204458589474597829394042491912841796875]
      mask Display: e = 0.06;c1 = [120 150 230]/255;c2 = ([120 150 230]+0)/383;c3 = ([120 150 230]+128)/383;patch([0 1 1 0],[0 0 1 1],c1);patch([0 1 1 1-e 1-e 0+e],[0 0 1 1-e 0+e 0+e],c2);patch([0 0 1 1-e 0+e 0+e],[0 1 1 1-e 1-e 0+e],c3);plot([0 1 1 0 0],[0 0 1 1 0]);disp('b');
  netsum : Sum  Inputs=2  SaturateOnIntegerOverflow=on  InputSameDT=on  OutDataTypeStr=Inherit: Same as first input
      mask Display: e = 0.06;c1 = [120 150 230]/255;c2 = ([120 150 230]+0)/383;c3 = ([120 150 230]+128)/383;patch([0 1 1 0],[0 0 1 1],c1);patch([0 1 1 1-e 1-e 0+e],[0 0 1 1-e 0+e 0+e],c2);patch([0 0 1 1-e 0+e 0+e],[0 1 1 1-e 1-e 0+e],c3);plot([0 1 1 0 0],[0 0 1 1 0]);disp('+');
  tansig : neural/Transfer Functions/tansig
      settings: SourceProductName=Deep Learning Toolbox
  "a{6}" : Outport  InitialOutput=[0;0;0;0;0;0;0;0;0;0;0;0;0;0;0;0;0;0;0;0;0;0;0;0;0;0;0;0;0;0;0;0;0;0;0;0;0;0;0;0;0;0;0;0;0;0;0;0;0;0]
      mask Display: e = 0.06;c1 = [120 230 180]/255;c2 = ([120 230 180]+0)/(256+128);c3 = ([120 230 180]+128)/(256+128);patch([0 1 1 0],[0 0 1 1],c1);patch([0 1 1 1-e 1-e 0+e],[0 0 1 1-e 0+e 0+e],c2);patch([0 0 1 1-e 0+e 0+e],[0 1 1 1-e 1-e 0+e],c3);plot([0 1 1 0 0],[0 0 1 1 0]);
  wires:
  tansig/1 -> "a{6}"/1
  netsum/1 -> tansig/1
  "b{6}"/1 -> netsum/2
  "LW{6,5}"/1("lz{6,5}") -> netsum/1
  Delays 1/1("pd{6,5}") -> "LW{6,5}"/1("ad{6,5}")
  "a{5} "/1 -> Delays 1/1("p{6}")

== system AcasXuClosedLoop_m_1/networks/AcasXu_3_1/Layer 7 ==
  "a{6} " : Inport  PortDimensions=50
      mask Display: e = 0.06;c1 = [120 230 180]/255;c2 = ([120 230 180]+0)/(256+128);c3 = ([120 230 180]+128)/(256+128);patch([0 1 1 0],[0 0 1 1],c1);patch([0 1 1 1-e 1-e 0+e],[0 0 1 1-e 0+e 0+e],c2);patch([0 0 1 1-e 0+e 0+e],[0 1 1 1-e 1-e 0+e],c3);plot([0 1 1 0 0],[0 0 1 1 0]);
  Delays 1 : Subsystem
      mask Display: e = 0.06;c1 = [120 150 230]/255;c2 = ([120 150 230]+0)/383;c3 = ([120 150 230]+128)/383;patch([0 1 1 0],[0 0 1 1],c1);patch([0 1 1 1-e 1-e 0+e],[0 0 1 1-e 0+e 0+e],c2);patch([0 0 1 1-e 0+e 0+e],[0 1 1 1-e 1-e 0+e],c3);plot([0 1 1 0 0],[0 0 1 1 0]);disp('0');
  "LW{7,6}" : Subsystem
      mask Display: e = 0.06;c1 = [120 150 230]/255;c2 = ([120 150 230]+0)/383;c3 = ([120 150 230]+128)/383;patch([0 1 1 0],[0 0 1 1],c1);patch([0 1 1 1-e 1-e 0+e],[0 0 1 1-e 0+e 0+e],c2);patch([0 0 1 1-e 0+e 0+e],[0 1 1 1-e 1-e 0+e],c3);plot([0 1 1 0 0],[0 0 1 1 0]);disp('W');
  "b{7}" : Constant  Value=[0.07839839999999999309299170136000611819326877593994140625;0.0810950000000000004174438572590588591992855072021484375;0.038134200000000000041477932199995848350226879119873046875;0.07972369999999999456985477763737435452640056610107421875;0.0160229999999999990489829571060909074731171131134033203125]
      mask Display: e = 0.06;c1 = [120 150 230]/255;c2 = ([120 150 230]+0)/383;c3 = ([120 150 230]+128)/383;patch([0 1 1 0],[0 0 1 1],c1);patch([0 1 1 1-e 1-e 0+e],[0 0 1 1-e 0+e 0+e],c2);patch([0 0 1 1-e 0+e 0+e],[0 1 1 1-e 1-e 0+e],c3);plot([0 1 1 0 0],[0 0 1 1 0]);disp('b');
  netsum : Sum  Inputs=2  SaturateOnIntegerOverflow=on  InputSameDT=on  OutDataTypeStr=Inherit: Same as first input
      mask Display: e = 0.06;c1 = [120 150 230]/255;c2 = ([120 150 230]+0)/383;c3 = ([120 150 230]+128)/383;patch([0 1 1 0],[0 0 1 1],c1);patch([0 1 1 1-e 1-e 0+e],[0 0 1 1-e 0+e 0+e],c2);patch([0 0 1 1-e 0+e 0+e],[0 1 1 1-e 1-e 0+e],c3);plot([0 1 1 0 0],[0 0 1 1 0]);disp('+');
  purelin : neural/Transfer Functions/purelin
      settings: SourceProductName=Deep Learning Toolbox
  "a{7}" : Outport  InitialOutput=[0;0;0;0;0]
      mask Display: e = 0.06;c1 = [120 230 180]/255;c2 = ([120 230 180]+0)/(256+128);c3 = ([120 230 180]+128)/(256+128);patch([0 1 1 0],[0 0 1 1],c1);patch([0 1 1 1-e 1-e 0+e],[0 0 1 1-e 0+e 0+e],c2);patch([0 0 1 1-e 0+e 0+e],[0 1 1 1-e 1-e 0+e],c3);plot([0 1 1 0 0],[0 0 1 1 0]);
  wires:
  purelin/1 -> "a{7}"/1
  netsum/1 -> purelin/1
  "b{7}"/1 -> netsum/2
  "LW{7,6}"/1("lz{7,6}") -> netsum/1
  Delays 1/1("pd{7,6}") -> "LW{7,6}"/1("ad{7,6}")
  "a{6} "/1 -> Delays 1/1("p{7}")

== system AcasXuClosedLoop_m_1/networks/AcasXu_3_1/Process Input 1 ==
  x : Inport  PortDimensions=5
      mask Display: e = 0.06;c1 = [120 230 180]/255;c2 = ([120 230 180]+0)/(256+128);c3 = ([120 230 180]+128)/(256+128);patch([0 1 1 0],[0 0 1 1],c1);patch([0 1 1 1-e 1-e 0+e],[0 0 1 1-e 0+e 0+e],c2);patch([0 0 1 1-e 0+e 0+e],[0 1 1 1-e 1-e 0+e],c3);plot([0 1 1 0 0],[0 0 1 1 0]);
  p : Outport  PortDimensions=5
      mask Display: e = 0.06;c1 = [120 230 180]/255;c2 = ([120 230 180]+0)/(256+128);c3 = ([120 230 180]+128)/(256+128);patch([0 1 1 0],[0 0 1 1],c1);patch([0 1 1 1-e 1-e 0+e],[0 0 1 1-e 0+e 0+e],c2);patch([0 0 1 1-e 0+e 0+e],[0 1 1 1-e 1-e 0+e],c3);plot([0 1 1 0 0],[0 0 1 1 0]);
  wires:
  x/1 -> p/1

== system AcasXuClosedLoop_m_1/networks/AcasXu_3_1/Process Output 1 ==
  a : Inport  PortDimensions=5
      mask Display: e = 0.06;c1 = [120 230 180]/255;c2 = ([120 230 180]+0)/(256+128);c3 = ([120 230 180]+128)/(256+128);patch([0 1 1 0],[0 0 1 1],c1);patch([0 1 1 1-e 1-e 0+e],[0 0 1 1-e 0+e 0+e],c2);patch([0 0 1 1-e 0+e 0+e],[0 1 1 1-e 1-e 0+e],c3);plot([0 1 1 0 0],[0 0 1 1 0]);
  y : Outport  PortDimensions=5
      mask Display: e = 0.06;c1 = [120 230 180]/255;c2 = ([120 230 180]+0)/(256+128);c3 = ([120 230 180]+128)/(256+128);patch([0 1 1 0],[0 0 1 1],c1);patch([0 1 1 1-e 1-e 0+e],[0 0 1 1-e 0+e 0+e],c2);patch([0 0 1 1-e 0+e 0+e],[0 1 1 1-e 1-e 0+e],c3);plot([0 1 1 0 0],[0 0 1 1 0]);
  wires:
  a/1 -> y/1

== system AcasXuClosedLoop_m_1/networks/AcasXu_4_1/Layer 1 ==
  "p{1}" : Inport  PortDimensions=5
      mask Display: e = 0.06;c1 = [120 230 180]/255;c2 = ([120 230 180]+0)/(256+128);c3 = ([120 230 180]+128)/(256+128);patch([0 1 1 0],[0 0 1 1],c1);patch([0 1 1 1-e 1-e 0+e],[0 0 1 1-e 0+e 0+e],c2);patch([0 0 1 1-e 0+e 0+e],[0 1 1 1-e 1-e 0+e],c3);plot([0 1 1 0 0],[0 0 1 1 0]);
  Delays 1 : Subsystem
      mask Display: e = 0.06;c1 = [120 150 230]/255;c2 = ([120 150 230]+0)/383;c3 = ([120 150 230]+128)/383;patch([0 1 1 0],[0 0 1 1],c1);patch([0 1 1 1-e 1-e 0+e],[0 0 1 1-e 0+e 0+e],c2);patch([0 0 1 1-e 0+e 0+e],[0 1 1 1-e 1-e 0+e],c3);plot([0 1 1 0 0],[0 0 1 1 0]);disp('0');
  "IW{1,1}" : Subsystem
      mask Display: e = 0.06;c1 = [120 150 230]/255;c2 = ([120 150 230]+0)/383;c3 = ([120 150 230]+128)/383;patch([0 1 1 0],[0 0 1 1],c1);patch([0 1 1 1-e 1-e 0+e],[0 0 1 1-e 0+e 0+e],c2);patch([0 0 1 1-e 0+e 0+e],[0 1 1 1-e 1-e 0+e],c3);plot([0 1 1 0 0],[0 0 1 1 0]);disp('W');
  "b{1}" : Constant  Value=[0.1348229999999999983995024877003743313252925872802734375;-0.0238180999999999983007814563507054117508232593536376953125;-0.11955000000000000348610029732299153693020343780517578125;-0.380141000000000006675549002466141246259212493896484375;-0.453220000000000011741718708435655571520328521728515625;-0.7901599999999999734967559561482630670070648193359375;-0.59201899999999996193622564533143304288387298583984375;-0.060997400000000000230837571280062547884881496429443359375;0.041191899999999996573318838954946841113269329071044921875;0.138994000000000006433964472307707183063030242919921875;0.5230390000000000316759951601852662861347198486328125;0.1683389999999999886437507257141987793147563934326171875;-0.2097199999999999897593028208575560711324214935302734375;-0.30047699999999999409538986583356745541095733642578125;-0.6601470000000000393214349969639442861080169677734375;0.33775800000000000267164068645797669887542724609375;-0.72938300000000000355981910615810193121433258056640625;-0.354287999999999991818100397722446359694004058837890625;0.330224000000000017518431150165270082652568817138671875;-0.01135309999999999965025754278258318663574755191802978515625;-0.0360036999999999995925037410415825434029102325439453125;-0.0244249999999999987954080182817051536403596401214599609375;0.2328119999999999911732828650201554410159587860107421875;0.1819800000000000028688162956314045004546642303466796875;0.03522630000000000205506722750214976258575916290283203125;0.45888200000000001210764821735210716724395751953125;-0.178321000000000007279510327862226404249668121337890625;0.055081100000000000893596308060295996256172657012939453125;-0.01507080000000000051529891464952015667222440242767333984375;-0.4580159999999999786979287819121964275836944580078125;-0.0500089999999999978985698589895037002861499786376953125;0.06709189999999999598490063590361387468874454498291015625;-0.323990999999999973457676105681457556784152984619140625;0.233887000000000011556977597138029523193836212158203125;0.1795219999999999871409528395815868861973285675048828125;-0.47103499999999998149036173344939015805721282958984375;0.11780400000000000593214366517713642679154872894287109375;-0.1605830000000000035154101851730956695973873138427734375;-0.02595340000000000146851419913218705914914608001708984375;-0.19649199999999999999289457264239899814128875732421875;0.09367630000000000400905975084242527373135089874267578125;-0.264062999999999992173371765602496452629566192626953125;-0.350741000000000024972024448288721032440662384033203125;-0.68448200000000003484501576167531311511993408203125;-0.2153859999999999941255879321033717133104801177978515625;0.60005299999999994753352439147420227527618408203125;0.276144000000000000571986902286880649626255035400390625;-0.57574000000000002952305067083216272294521331787109375;-0.5823739999999999472635181518853642046451568603515625;0.1123949999999999949107376551182824186980724334716796875]
      mask Display: e = 0.06;c1 = [120 150 230]/255;c2 = ([120 150 230]+0)/383;c3 = ([120 150 230]+128)/383;patch([0 1 1 0],[0 0 1 1],c1);patch([0 1 1 1-e 1-e 0+e],[0 0 1 1-e 0+e 0+e],c2);patch([0 0 1 1-e 0+e 0+e],[0 1 1 1-e 1-e 0+e],c3);plot([0 1 1 0 0],[0 0 1 1 0]);disp('b');
  netsum : Sum  Inputs=2  SaturateOnIntegerOverflow=on  InputSameDT=on  OutDataTypeStr=Inherit: Same as first input
      mask Display: e = 0.06;c1 = [120 150 230]/255;c2 = ([120 150 230]+0)/383;c3 = ([120 150 230]+128)/383;patch([0 1 1 0],[0 0 1 1],c1);patch([0 1 1 1-e 1-e 0+e],[0 0 1 1-e 0+e 0+e],c2);patch([0 0 1 1-e 0+e 0+e],[0 1 1 1-e 1-e 0+e],c3);plot([0 1 1 0 0],[0 0 1 1 0]);disp('+');
  tansig : neural/Transfer Functions/tansig
      settings: SourceProductName=Deep Learning Toolbox
  "a{1}" : Outport  InitialOutput=[0;0;0;0;0;0;0;0;0;0;0;0;0;0;0;0;0;0;0;0;0;0;0;0;0;0;0;0;0;0;0;0;0;0;0;0;0;0;0;0;0;0;0;0;0;0;0;0;0;0]
      mask Display: e = 0.06;c1 = [120 230 180]/255;c2 = ([120 230 180]+0)/(256+128);c3 = ([120 230 180]+128)/(256+128);patch([0 1 1 0],[0 0 1 1],c1);patch([0 1 1 1-e 1-e 0+e],[0 0 1 1-e 0+e 0+e],c2);patch([0 0 1 1-e 0+e 0+e],[0 1 1 1-e 1-e 0+e],c3);plot([0 1 1 0 0],[0 0 1 1 0]);
  wires:
  tansig/1 -> "a{1}"/1
  netsum/1 -> tansig/1
  "b{1}"/1 -> netsum/2
  "IW{1,1}"/1("iz{1,1}") -> netsum/1
  Delays 1/1("pd{1,1}") -> "IW{1,1}"/1("pd{1,1}")
  "p{1}"/1 -> Delays 1/1("p{1}")

== system AcasXuClosedLoop_m_1/networks/AcasXu_4_1/Layer 2 ==
  "a{1} " : Inport  PortDimensions=50
      mask Display: e = 0.06;c1 = [120 230 180]/255;c2 = ([120 230 180]+0)/(256+128);c3 = ([120 230 180]+128)/(256+128);patch([0 1 1 0],[0 0 1 1],c1);patch([0 1 1 1-e 1-e 0+e],[0 0 1 1-e 0+e 0+e],c2);patch([0 0 1 1-e 0+e 0+e],[0 1 1 1-e 1-e 0+e],c3);plot([0 1 1 0 0],[0 0 1 1 0]);
  Delays 1 : Subsystem
      mask Display: e = 0.06;c1 = [120 150 230]/255;c2 = ([120 150 230]+0)/383;c3 = ([120 150 230]+128)/383;patch([0 1 1 0],[0 0 1 1],c1);patch([0 1 1 1-e 1-e 0+e],[0 0 1 1-e 0+e 0+e],c2);patch([0 0 1 1-e 0+e 0+e],[0 1 1 1-e 1-e 0+e],c3);plot([0 1 1 0 0],[0 0 1 1 0]);disp('0');
  "LW{2,1}" : Subsystem
      mask Display: e = 0.06;c1 = [120 150 230]/255;c2 = ([120 150 230]+0)/383;c3 = ([120 150 230]+128)/383;patch([0 1 1 0],[0 0 1 1],c1);patch([0 1 1 1-e 1-e 0+e],[0 0 1 1-e 0+e 0+e],c2);patch([0 0 1 1-e 0+e 0+e],[0 1 1 1-e 1-e 0+e],c3);plot([0 1 1 0 0],[0 0 1 1 0]);disp('W');
  "b{2}" : Constant  Value=[0.432821999999999984520826501466217450797557830810546875;-1.259370000000000100470742836478166282176971435546875;-0.45713700000000001555378048578859306871891021728515625;-0.65248300000000003517897084748256020247936248779296875;0.0116892000000000002846167745929051307030022144317626953125;0.9686099999999999710098563809879124164581298828125;-0.00109700000000000010176581799470341138658113777637481689453125;-0.01449650000000000070465855372958685620687901973724365234375;-0.01553530000000000015070167336261874879710376262664794921875;-0.1711300000000000043343106881366111338138580322265625;1.346410000000000106723518911167047917842864990234375;-0.0236382000000000015715873047383865923620760440826416015625;1.136740000000000083701934272539801895618438720703125;-0.98688699999999995871036162498057819902896881103515625;-0.202730999999999994543031789362430572509765625;0.28883599999999998164668113531661219894886016845703125;-0.18953900000000001302424834648263640701770782470703125;-0.67643200000000003324629460621508769690990447998046875;-0.77303200000000005243094847173779271543025970458984375;1.2642599999999999393907046396634541451930999755859375;-0.51136499999999995846877709482214413583278656005859375;1.3603799999999999226218960757250897586345672607421875;-0.0432717999999999991533883303418406285345554351806640625;-0.273573999999999983856469043530523777008056640625;0.3089749999999999996447286321199499070644378662109375;-0.05264359999999999872866141004124074243009090423583984375;1.1708000000000000628830321147688664495944976806640625;-0.01064329999999999963600227914639617665670812129974365234375;-0.50644199999999994776800349427503533661365509033203125;0.1564000000000000112354570092065841890871524810791015625;0.1855920000000000069650951672883820720016956329345703125;-0.0237028999999999989700683045157347805798053741455078125;-0.95172800000000001841016228354419581592082977294921875;-0.322857000000000005091038701721117831766605377197265625;-0.382485000000000019415580254644737578928470611572265625;-0.1345760000000000011777245845223660580813884735107421875;-0.01455150000000000019839685450051547377370297908782958984375;-0.269760999999999973031350464225397445261478424072265625;-0.88523399999999996534683077697991393506526947021484375;9.9680700000000002614607141904201625948189757764339447021484375e-05;-0.0100038999999999995982324918486483511514961719512939453125;1.2512399999999999078426071719150058925151824951171875;0.171111999999999986332710477654472924768924713134765625;-0.409106000000000025185187269016751088201999664306640625;-0.6994439999999999546531626037904061377048492431640625;0.444589999999999985202947527795913629233837127685546875;0.535841000000000011738165994756855070590972900390625;0.04694199999999999761701729994456400163471698760986328125;0.2113869999999999915729631538852117955684661865234375;0.58456699999999994776800349427503533661365509033203125]
      mask Display: e = 0.06;c1 = [120 150 230]/255;c2 = ([120 150 230]+0)/383;c3 = ([120 150 230]+128)/383;patch([0 1 1 0],[0 0 1 1],c1);patch([0 1 1 1-e 1-e 0+e],[0 0 1 1-e 0+e 0+e],c2);patch([0 0 1 1-e 0+e 0+e],[0 1 1 1-e 1-e 0+e],c3);plot([0 1 1 0 0],[0 0 1 1 0]);disp('b');
  netsum : Sum  Inputs=2  SaturateOnIntegerOverflow=on  InputSameDT=on  OutDataTypeStr=Inherit: Same as first input
      mask Display: e = 0.06;c1 = [120 150 230]/255;c2 = ([120 150 230]+0)/383;c3 = ([120 150 230]+128)/383;patch([0 1 1 0],[0 0 1 1],c1);patch([0 1 1 1-e 1-e 0+e],[0 0 1 1-e 0+e 0+e],c2);patch([0 0 1 1-e 0+e 0+e],[0 1 1 1-e 1-e 0+e],c3);plot([0 1 1 0 0],[0 0 1 1 0]);disp('+');
  tansig : neural/Transfer Functions/tansig
      settings: SourceProductName=Deep Learning Toolbox
  "a{2}" : Outport  InitialOutput=[0;0;0;0;0;0;0;0;0;0;0;0;0;0;0;0;0;0;0;0;0;0;0;0;0;0;0;0;0;0;0;0;0;0;0;0;0;0;0;0;0;0;0;0;0;0;0;0;0;0]
      mask Display: e = 0.06;c1 = [120 230 180]/255;c2 = ([120 230 180]+0)/(256+128);c3 = ([120 230 180]+128)/(256+128);patch([0 1 1 0],[0 0 1 1],c1);patch([0 1 1 1-e 1-e 0+e],[0 0 1 1-e 0+e 0+e],c2);patch([0 0 1 1-e 0+e 0+e],[0 1 1 1-e 1-e 0+e],c3);plot([0 1 1 0 0],[0 0 1 1 0]);
  wires:
  tansig/1 -> "a{2}"/1
  netsum/1 -> tansig/1
  "b{2}"/1 -> netsum/2
  "LW{2,1}"/1("lz{2,1}") -> netsum/1
  Delays 1/1("pd{2,1}") -> "LW{2,1}"/1("ad{2,1}")
  "a{1} "/1 -> Delays 1/1("p{2}")
